simulink model "prbs_6bits"  (Simulink 6.6)
settings: Solver=FixedStepDiscrete  StartTime=0.0  StopTime=63  FixedStep=1  RelTol=1e-3
undefined symbols (not defined in the file): TS_PRBS
settings Model: Creator=bailly  LastModifiedBy=bailly

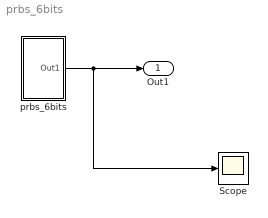
== system prbs_6bits ==
  Scope : Scope
  prbs_6bits : Subsystem
  Out1 : Outport
  wires:
  prbs_6bits/1(Out1) -> Out1/1, Scope/1

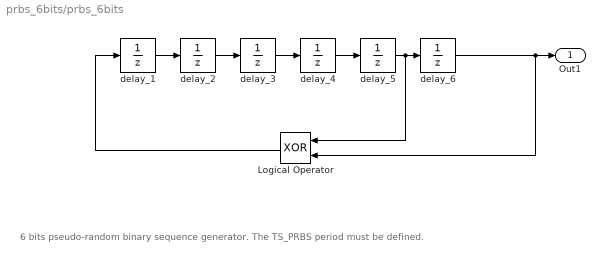
== system prbs_6bits/prbs_6bits ==
  note: 6 bits pseudo-random binary sequence generator.
      | The TS_PRBS period must be defined.
  Logical Operator : Logic  Orientation=left  Operator=XOR  AllPortsSameDT=off  OutDataTypeMode=Boolean
  delay_1 : UnitDelay  X0=1  SampleTime=TS_PRBS
  delay_{2..6} (5 alike) : UnitDelay  X0=1  SampleTime=-1
  Out1 : Outport
  wires:
  delay_5/1 -> delay_6/1, Logical Operator/1
  delay_6/1 -> Logical Operator/2, Out1/1
  delay_2/1 -> delay_3/1
  delay_3/1 -> delay_4/1
  delay_4/1 -> delay_5/1
  delay_1/1 -> delay_2/1
  Logical Operator/1 -> delay_1/1
